simulink subsystem "Transformada_Directa_de_Park_I"  (R2026a)
settings: Solver=VariableStepAuto
values from neighbouring files (symbols this model uses):
  Pp = 3    [coeficientes.m]
libraries: eeTransforms x1
settings Model: Creator=admin  LastModifiedBy=admin

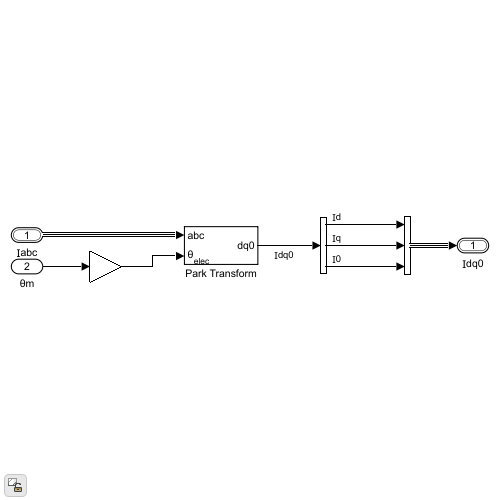
[thumbnail: Simulink's stored preview of the top-level diagram]
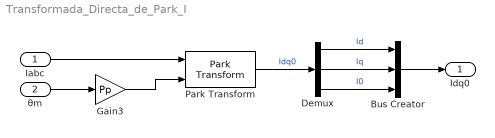
== system Transformada_Directa_de_Park_I ==
  Ⅰabc : Inport  OutDataTypeStr=Bus: Iabc
  θm : Inport  Port=2
  Bus Creator : BusCreator  Inputs=3
  Demux : Demux  Outputs=3
  Gain3 : Gain  Gain=Pp
  Park Transform : eeTransforms/Park Transform  AxisAlignment=Q-axis  PowerInvariant=off
      settings: LibrarySourceBlock=|
      | ee_sl_lib/Mathematical
      | Transforms/Park Transform
  Ⅰdq0 : Outport  OutDataTypeStr=Bus: Idq0
  wires:
  Gain3/1 -> Park Transform/2
  Park Transform/1 -> Demux/1  "Ⅰdq0"
  Demux/1 -> Bus Creator/1  "Ⅰd"
  Demux/3 -> Bus Creator/3  "Ⅰ0"
  Demux/2 -> Bus Creator/2  "Ⅰq"
  Bus Creator/1 -> Ⅰdq0/1
  Ⅰabc/1 -> Park Transform/1
  θm/1 -> Gain3/1
